simulink model "recepteur_emetteur_uspr"  (R2017a)
settings: Solver=VariableStepAuto  StartTime=0.0  StopTime=inf  RelTol=1e-3
libraries: commsdrhw_v2 x1
settings Model: Creator=max  LastModifiedBy=max
settings DataIOCC: LimitDataPoints=on  SaveOutput=off  SaveTime=off
settings OptimizationCC: BlockReduction=off  BooleanDataType=off  LifeSpan=inf
settings DebuggingCC: SaveWithParameterizedLinksMsg=none  UnderspecifiedInitializationDetection=Classic  MergeDetectMultiDrivingBlocksExec=none  SignalResolutionControl=TryResolveAllWithWarning  AllowSymbolicDim=off  SFUnexpectedBacktrackingDiag=warning  SFNoUnconditionalDefaultTransitionDiag=warning  SFExecutionAtInitializationDiag=none
settings HardwareCC: TargetUnknown=on
settings GRTTargetCC: TargetLangStandard=C89/C90 (ANSI)  GeneratePreprocessorConditionals=Disable all

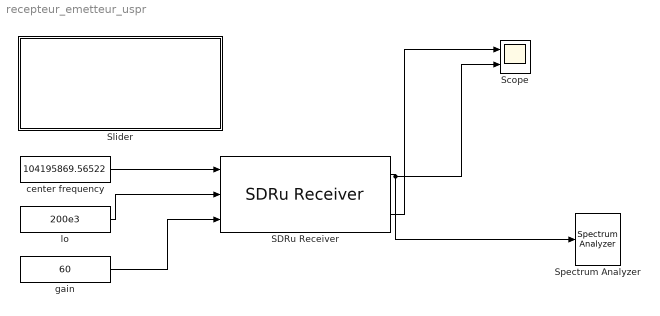
== system recepteur_emetteur_uspr ==
  SDRu Receiver : commsdrhw_v2/SDRu Receiver  SourceLibraryInfo="This block requires <a href=\"http://www.mathworks.com/hardware-support/usrp.html\">Communications System Toolbox Support Package for USRP Radio</a>"  rxtx=rx  platform=B210  USRP2_IP='192.168.10.2'  USRP_IP_X300='192.168.10.2'  USRP_IP_X310='192.168.10.2'  USRP_serialNumB200=''  USRP_serialNumB210='30CEEA7'  ChannelMapping=1  centerFrequency=93294130.434783  centerFrequencySrc=Input port  loOffset=200  loOffsetSrc=Input port  PPSSource=Internal  clockSource=Internal  masterClkRateB200=32e6  masterClkRateB210=32e6  masterClkRateX300=200e6  masterClkRateX310=200e6  masterClkRateParam=32000000  gain=60  gainSrc=Input port  decimInterpSrc=Dialog  decimInterp=16  TransportDataType=int16  USRP2_IP_NUM=[51 48 67 69 69 65 55]  frameLength=4096  outputDatatype=Same as transport data type  overrunUnderrunPort=off  sampleTime=1/2e6  HOST_DATA_PORT=0  HOST_CONTROL_PORT=0  USRP2_DATA_PORT=0  USRP2_CONTROL_PORT=0  bufferMode=Continuous streaming  EnableBurstMode=off  NumFramesInBurst=100  USRP_ID='30CEEA7'
      settings: SourceProductName=Communications System Toolbox Support Package for USRP(R) Radio  SourceProductBaseCode=USRP
  Scope : Scope  NumInputPorts=2
  Slider : Subsystem  DialogController=hmiCreateDDGDialog  IsWebBlock=on  mask(MWDashboardBlock){webBlockId=15bf7502-6270-4803-a67f-b5dded809f6e, webBlockType=slider, ShowInLibBrowser=on, ShowInitialText=on, HMISrcModelName=recepteur_radio_fm_uspr}
      mask prompts: webBlockId "WebBlock Id"; webBlockType "WebBlock Type"; HMISrcModelName "Source Model"
      mask help: SimulinkHMI:dialogs:SliderDialogDesc
      mask Help: helpview([docroot '/mapfiles/simulink.map'], 'hmi_slider')
      mask Display:
      | if strcmp(get_param(bdroot(gcb),'BlockDiagramType'), 'library')
      |     image([(matlabroot) '/toolbox/simulink/hmi/icons/Slider.png']);
      | end
  Spectrum Analyzer : SpectrumAnalyzer
  center frequency : Constant  Value=104195869.56522
  "gain " : Constant  Value=60
  lo : Constant  Value=200e3
  wires:
  SDRu Receiver/1 -> Scope/2, Spectrum Analyzer/1
  SDRu Receiver/2 -> Scope/1
  "gain "/1 -> SDRu Receiver/3
  lo/1 -> SDRu Receiver/2
  center frequency/1 -> SDRu Receiver/1

== system recepteur_emetteur_uspr/Slider ==
